simulink model "G_block"  (R2020a)
settings: Solver=VariableStepAuto  StartTime=0.0  StopTime=10.0  RelTol=1e-3
undefined symbols (not defined in the file): g, l1, lc1, lc2, m1, m2
settings Model: Creator=fernando  LastModifiedBy=fernando

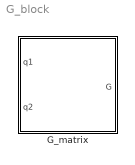
== system G_block ==
  G_matrix : MATLAB Function  TreatAsAtomicUnit=on

== matlab function G_block/G_matrix ==
  data: G output; q1 input; q2 input; g parameter; l1 parameter; lc1 parameter; lc2 parameter; m1 parameter; m2 parameter
function G = G_matrix(q1,q2, g, l1, lc1, lc2, m1, m2)
%#codegen

%    This function was generated by the Symbolic Math Toolbox version 8.3.
%    05-Nov-2019 15:18:30

t2 = cos(q1);
t3 = q1+q2;
t4 = cos(t3);
G = [g.*m2.*(l1.*t2+lc2.*t4)+g.*lc1.*m1.*t2;g.*lc2.*m2.*t4];
